simulink model "hbridge_inverter_lc_closed_loop"  (R2025b)
settings: Solver=ode3  StartTime=0.0  StopTime=T_sim_control  FixedStep=T_step  RelTol=1e-3
values from neighbouring files (symbols this model uses):
  C_f = 47e-6    (= 4.7e-05)    [inverter_params.m]
  Ki_voltage = 1.20    (= 1.2)    [inverter_params.m]
  Kp_voltage = 0.010    (= 0.01)    [inverter_params.m]
  L_f = 100e-6    (= 0.0001)    [inverter_params.m]
  m_max = 0.95    [inverter_params.m]
  m_min = 0.00    (= 0)    [inverter_params.m]
  N_line_cycle = round(1 / (f_grid * T_step))    [inverter_params.m]
  omega_0 = 2 * pi * f_grid    (= 314.159265359)    [inverter_params.m]
  R_d_total = R_d + R_Cf_esr    (= 0.51)    [inverter_params.m]
  R_Lf = 0.015    [inverter_params.m]
  R_load_half = (V_out_rms_ref^2) / (0.5 * P_nom)    [inverter_params.m]
  R_load_nom = (V_out_rms_ref^2) / P_nom    [inverter_params.m]
  t_load_step = 0.18    [inverter_params.m]
  t_soft_start = 0.06    [inverter_params.m]
  T_step = 1e-6    (= 1e-06)    [inverter_params.m]
  V_out_pk_ref = sqrt(2) * V_out_rms_ref    [inverter_params.m]
  Vdc = 48.0    (= 48)    [inverter_params.m]
undefined symbols (not defined in the file or in its folder): DiscIntNeverNeededParam
libraries: simulink x2
settings Model: Creator=hemanggadhvi  LastModifiedBy=hemanggadhvi

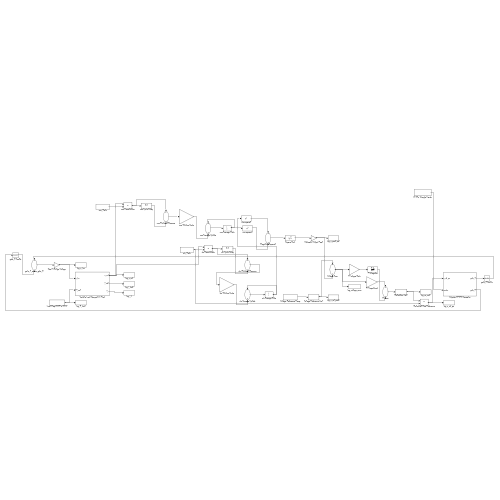
[thumbnail: Simulink's stored preview of the top-level diagram]
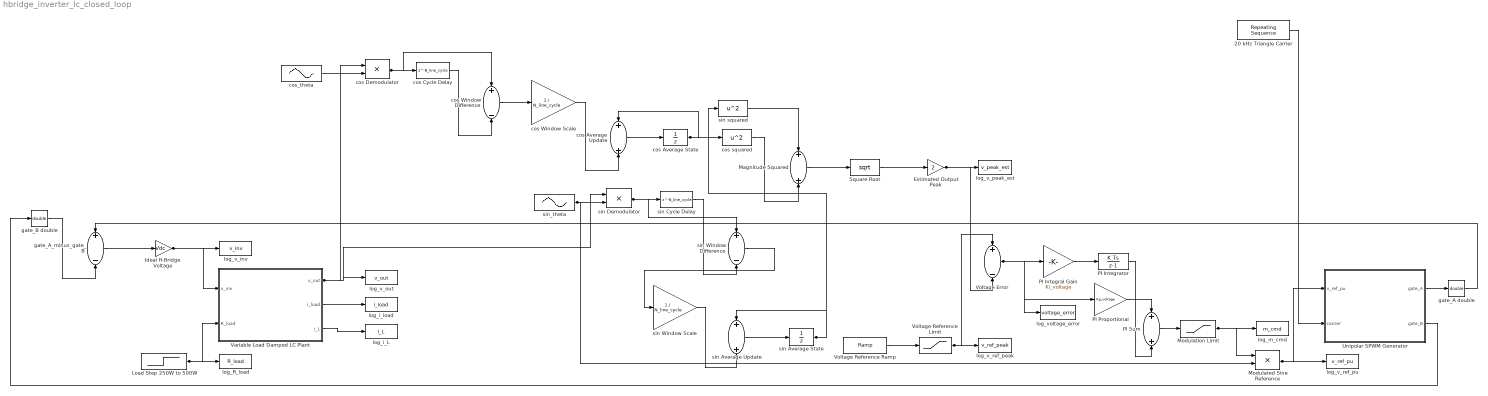
== system hbridge_inverter_lc_closed_loop ==
  20 kHz Triangle Carrier : simulink/Sources/Repeating Sequence  rep_seq_t=carrier_time  rep_seq_y=carrier_values
  Estimated Output Peak : Gain  Gain=2
  Ideal H-Bridge Voltage : Gain  Gain=Vdc
  Load Step 250W to 500W : Step  Time=t_load_step  Before=R_load_half  After=R_load_nom  SampleTime=0
  Magnitude Squared : Sum
  Modulated Sine Reference : Product
  Modulation Limit : Saturate  UpperLimit=m_max  LowerLimit=m_min
  PI Integral Gain : Gain  Gain=Ki_voltage
  PI Integrator : DiscreteIntegrator  SampleTime=T_step  ICPrevOutput=DiscIntNeverNeededParam  ICPrevScaledInput=DiscIntNeverNeededParam
  PI Proportional : Gain  Gain=Kp_voltage
  PI Sum : Sum
  Square Root : Math  Operator=sqrt
  Unipolar SPWM Generator : Subsystem
  Variable Load Damped LC Plant : Subsystem
  Voltage Error : Sum  Inputs=+-
  Voltage Reference Limit : Saturate  UpperLimit=V_out_pk_ref  LowerLimit=0
  Voltage Reference Ramp : simulink/Sources/Ramp  slope=V_out_pk_ref / t_soft_start  start=0  InitialOutput=0
  cos Average State : UnitDelay  SampleTime=T_step  HasFrameUpgradeWarning=on
  cos Average Update : Sum
  cos Cycle Delay : Delay  DelayLength=N_line_cycle  InitialCondition=0  SampleTime=T_step
  cos Demodulator : Product
  cos Window Difference : Sum  Inputs=+-
  cos Window Scale : Gain  Gain=1 / N_line_cycle
  cos squared : Math  Operator=square
  cos_theta : Sin  Frequency=omega_0  Phase=pi/2  SampleTime=0
  gate_A double : DataTypeConversion  OutDataTypeStr=double  SaturateOnIntegerOverflow=off  RndMeth=Floor
  gate_A_minus_gate_B : Sum  Inputs=+-
  gate_B double : DataTypeConversion  OutDataTypeStr=double  SaturateOnIntegerOverflow=off  RndMeth=Floor
  log_R_load : ToWorkspace  VariableName=R_load  SaveFormat=Timeseries  SampleTime=-1
  log_i_L : ToWorkspace  VariableName=i_L  SaveFormat=Timeseries  SampleTime=-1
  log_i_load : ToWorkspace  VariableName=i_load  SaveFormat=Timeseries  SampleTime=-1
  log_m_cmd : ToWorkspace  VariableName=m_cmd  SaveFormat=Timeseries  SampleTime=-1
  log_v_inv : ToWorkspace  VariableName=v_inv  SaveFormat=Timeseries  SampleTime=-1
  log_v_out : ToWorkspace  VariableName=v_out  SaveFormat=Timeseries  SampleTime=-1
  log_v_peak_est : ToWorkspace  VariableName=v_peak_est  SaveFormat=Timeseries  SampleTime=-1
  log_v_ref_peak : ToWorkspace  VariableName=v_ref_peak  SaveFormat=Timeseries  SampleTime=-1
  log_v_ref_pu : ToWorkspace  VariableName=v_ref_pu  SaveFormat=Timeseries  SampleTime=-1
  log_voltage_error : ToWorkspace  VariableName=voltage_error  SaveFormat=Timeseries  SampleTime=-1
  sin Average State : UnitDelay  SampleTime=T_step  HasFrameUpgradeWarning=on
  sin Average Update : Sum
  sin Cycle Delay : Delay  DelayLength=N_line_cycle  InitialCondition=0  SampleTime=T_step
  sin Demodulator : Product
  sin Window Difference : Sum  Inputs=+-
  sin Window Scale : Gain  Gain=1 / N_line_cycle
  sin squared : Math  Operator=square
  sin_theta : Sin  Frequency=omega_0  SampleTime=0
  wires:
  Modulated Sine Reference/1 -> log_v_ref_pu/1, Unipolar SPWM Generator/1(v_ref_pu)
  20 kHz Triangle Carrier/1 -> Unipolar SPWM Generator/2(carrier)
  Modulation Limit/1 -> Modulated Sine Reference/1, log_m_cmd/1
  Unipolar SPWM Generator/1(gate_A) -> gate_A double/1
  PI Sum/1 -> Modulation Limit/1
  PI Proportional/1 -> PI Sum/1
  Voltage Reference Ramp/1 -> Voltage Reference Limit/1
  PI Integrator/1 -> PI Sum/2
  sin Average State/1 -> sin squared/1, sin Average Update/1
  Magnitude Squared/1 -> Square Root/1
  Voltage Error/1 -> log_voltage_error/1, PI Integral Gain/1, PI Proportional/1
  sin Average Update/1 -> sin Average State/1
  Voltage Reference Limit/1 -> log_v_ref_peak/1, Voltage Error/1
  sin Window Difference/1 -> sin Window Scale/1
  Variable Load Damped LC Plant/1(v_out) -> log_v_out/1, cos Demodulator/1, sin Demodulator/1
  sin Demodulator/1 -> sin Cycle Delay/1, sin Window Difference/1
  sin squared/1 -> Magnitude Squared/1
  sin Window Scale/1 -> sin Average Update/2
  Square Root/1 -> Estimated Output Peak/1
  sin Cycle Delay/1 -> sin Window Difference/2
  cos Average State/1 -> cos squared/1, cos Average Update/1
  Unipolar SPWM Generator/2(gate_B) -> gate_B double/1
  cos Average Update/1 -> cos Average State/1
  PI Integral Gain/1 -> PI Integrator/1
  sin_theta/1 -> sin Demodulator/2, Modulated Sine Reference/2
  Variable Load Damped LC Plant/2(i_load) -> log_i_load/1
  cos squared/1 -> Magnitude Squared/2
  cos Window Scale/1 -> cos Average Update/2
  cos Demodulator/1 -> cos Cycle Delay/1, cos Window Difference/1
  Variable Load Damped LC Plant/3(i_L) -> log_i_L/1
  Ideal H-Bridge Voltage/1 -> log_v_inv/1, Variable Load Damped LC Plant/1(v_inv)
  Load Step 250W to 500W/1 -> log_R_load/1, Variable Load Damped LC Plant/2(R_load)
  Estimated Output Peak/1 -> log_v_peak_est/1, Voltage Error/2
  cos Cycle Delay/1 -> cos Window Difference/2
  cos Window Difference/1 -> cos Window Scale/1
  gate_A_minus_gate_B/1 -> Ideal H-Bridge Voltage/1
  gate_A double/1 -> gate_A_minus_gate_B/1
  cos_theta/1 -> cos Demodulator/2
  gate_B double/1 -> gate_A_minus_gate_B/2

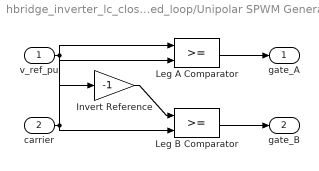
== system hbridge_inverter_lc_closed_loop/Unipolar SPWM Generator ==
  v_ref_pu : Inport
  carrier : Inport  Port=2
  Invert Reference : Gain  Gain=-1
  Leg A Comparator : RelationalOperator  OutDataTypeStr=boolean  RndMeth=Simplest  InputSameDT=off
  Leg B Comparator : RelationalOperator  OutDataTypeStr=boolean  RndMeth=Simplest  InputSameDT=off
  gate_A : Outport
  gate_B : Outport  Port=2
  wires:
  v_ref_pu/1 -> Leg A Comparator/1, Invert Reference/1
  carrier/1 -> Leg A Comparator/2, Leg B Comparator/2
  Invert Reference/1 -> Leg B Comparator/1
  Leg A Comparator/1 -> gate_A/1
  Leg B Comparator/1 -> gate_B/1

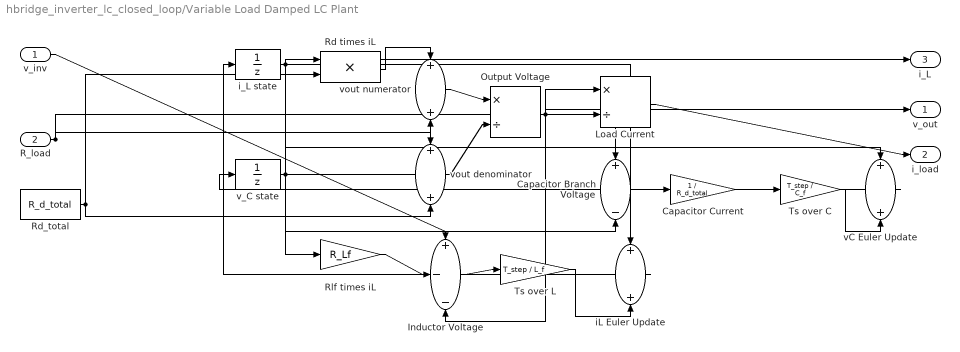
== system hbridge_inverter_lc_closed_loop/Variable Load Damped LC Plant ==
  v_inv : Inport
  R_load : Inport  Port=2
  Capacitor Branch Voltage : Sum  Inputs=+-
  Capacitor Current : Gain  Gain=1 / R_d_total
  Inductor Voltage : Sum  Inputs=+--
  Load Current : Product  Inputs=*/
  Output Voltage : Product  Inputs=*/
  Rd times iL : Product
  Rd_total : Constant  Value=R_d_total
  Rlf times iL : Gain  Gain=R_Lf
  Ts over C : Gain  Gain=T_step / C_f
  Ts over L : Gain  Gain=T_step / L_f
  iL Euler Update : Sum
  i_L state : UnitDelay  SampleTime=T_step  HasFrameUpgradeWarning=on
  vC Euler Update : Sum
  v_C state : UnitDelay  SampleTime=T_step  HasFrameUpgradeWarning=on
  vout denominator : Sum
  vout numerator : Sum
  v_out : Outport
  i_load : Outport  Port=2
  i_L : Outport  Port=3
  wires:
  i_L state/1 -> Rd times iL/1, Rlf times iL/1, iL Euler Update/1, i_L/1
  Rd_total/1 -> Rd times iL/2, vout denominator/2
  Rd times iL/1 -> vout numerator/1
  v_C state/1 -> vout numerator/2, Capacitor Branch Voltage/2, vC Euler Update/1
  R_load/1 -> vout denominator/1, Load Current/2
  vout numerator/1 -> Output Voltage/1
  vout denominator/1 -> Output Voltage/2
  Output Voltage/1 -> Load Current/1, Inductor Voltage/3, Capacitor Branch Voltage/1, v_out/1
  v_inv/1 -> Inductor Voltage/1
  Rlf times iL/1 -> Inductor Voltage/2
  Inductor Voltage/1 -> Ts over L/1
  Ts over L/1 -> iL Euler Update/2
  iL Euler Update/1 -> i_L state/1
  Capacitor Branch Voltage/1 -> Capacitor Current/1
  Capacitor Current/1 -> Ts over C/1
  Ts over C/1 -> vC Euler Update/2
  vC Euler Update/1 -> v_C state/1
  Load Current/1 -> i_load/1
